simulink model "mech_transmission"  (Simulink 7.1)
settings: Solver=ode45  StartTime=0.0  StopTime=100  RelTol=1e-4  AbsTol=1e-4
PreLoadFcn:
  | load mech_transmission_data;
undefined symbols (not defined in the file or in its folder): converter_data, downtab, emap, Iei, Iint, mutable, Nf, r1, r2, radvec, thvec, uptab, vehicledata
libraries: mblibv1 x64
(part 1 of 2)
Description:
  | Automobile Transmission
  | 
  | Detailed model of an automotive gear box with Stateflow logic.
  | 
  | Stateflow is required only if you want to modify the existing logic charts.
settings Model: Creator=The MathWorks Inc.  ExtModeAutoUpdateStatusClock=off  BufferReuse=off
settings DataIOCC: SaveState=on  SignalLoggingName=sigsOut
settings OptimizationCC: BooleanDataType=off  InlineInvariantSignals=on  OptimizeBlockIOStorage=off  BufferReuse=off  ExpressionFolding=off  LocalBlockOutputs=off
settings DebuggingCC: AlgebraicLoopMsg=none  SaveWithParameterizedLinksMsg=none  CheckExecutionContextPreStartOutputMsg=on  CheckExecutionContextRuntimeOutputMsg=on  SignalResolutionControl=TryResolveAllWithWarning  SolverPrmCheckMsg=none  MultiTaskDSMMsg=warning  MultiTaskCondExecSysMsg=none  SigSpecEnsureSampleTimeMsg=none  StrictBusMsg=None
settings HardwareCC: TargetBitPerLong=64  TargetEndianess=LittleEndian  TargetWordSize=64  TargetHWDeviceType=MATLAB Host  ProdEqTarget=off
settings RTWCC: SystemTargetFile=rsim.tlc  TemplateMakefile=rsim_default_tmf  Description=Rapid Simulation Target  ProcessScript=rsim_make_rtw_hook  IncludeERTFirstTime=on
settings RSimTargetCC: TargetFcnLib=ansi_tfl_tmw.mat  TargetFunctionLibrary=ANSI_C  IsPILTarget=off  EnableShiftOperators=on  PortableWordSizes=off

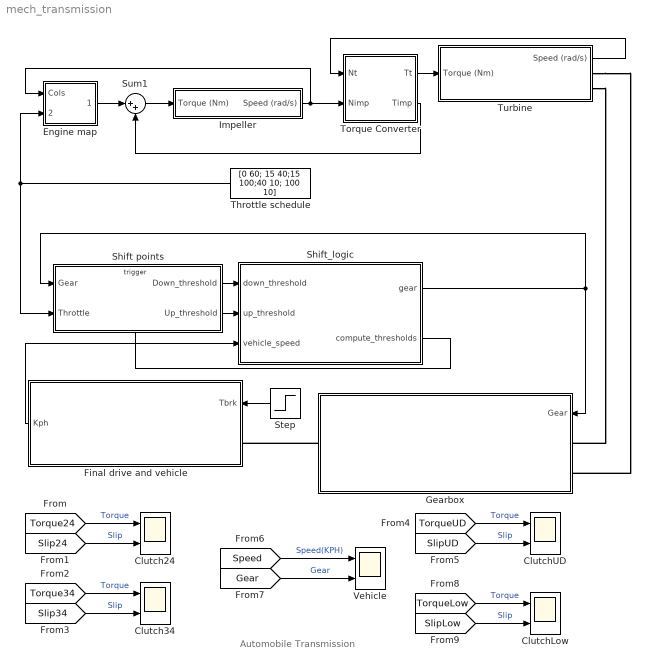
== system mech_transmission ==
  note: Automobile Transmission
  " Shift_logic" : Stateflow chart
  Clutch24 : Scope  NumInputPorts=2
      settings: TimeRange=100  YMin=-1000~-500  YMax=1000~500
  Clutch34 : Scope  NumInputPorts=2
      settings: TimeRange=100  YMin=-1000~-400  YMax=1000~200  SaveName=ScopeData2
  ClutchLow : Scope  NumInputPorts=2
      settings: TimeRange=100  YMin=-1000~0  YMax=500~600  SaveName=ScopeData4
  ClutchUD : Scope  NumInputPorts=2
      settings: TimeRange=100  YMin=-1000~-200  YMax=1000~400  SaveName=ScopeData3
  Engine map : Subsystem  AncestorBlock=|  mask(Lookup Table (2-D)){x=thvec, y=radvec, t=emap}
      | simulink3/Functions
      | & Tables/Look-Up
      | Table (2-D)
      mask prompts: x "Row:"; y "Column:"; t "Table:"
      mask help: Performs 2-D linear interpolation of input values using the specified input/output table. Extrapolation is performed outside the table boundaries. The first dimension corresponds to the top (or left) input port.
      mask init:
      | [r,c]=size(t);
      | xt=reshape(x,prod(size(x)),1);
      | xi=xt(:,ones(1,c));
      | minx=min(x); maxx=max(x);
      | mint=min(min(t)); maxt=max(max(t));
      mask Display: plot(double(xi),double(t),double([minx maxx]),double([mint mint]),double([minx minx]),double([mint maxt]))
  Final drive and vehicle : Subsystem  Orientation=left  mask(vehicle model){Rfd=vehicledata(1), rload0=vehicledata(2), rload2=vehicledata(3), Rw=vehicledata(4), inertiav=vehicledata(5), N20=vehicledata(6)/vehicledata(4)*vehicledata(1)}
      mask prompts: Rfd "Final drive ratio"; rload0 "Drag friction at wheels"; rload2 "Aerodynamic drag"; Rw "Wheel radius"; inertiav "Vehicle inertia"; N20 "Initial transmission output speed"
      mask help: vehicle dynamics: torque input from trans., outputs are input speed (transmission output) and vehicle speed
      mask Display: plot(-2,1,11,8,9-[cos(pi*[0:5:360]/180) + 6], [sin(pi*[0:5:360]/180) + 1.5],9-[cos(pi*[0:5:360]/180) + 1], [sin(pi*[0:5:360]/180) + 4],9- [10 7.5 6.75], [3.5 1 1.5], 9-[10 9.75 7.5 6.25 3 1.5 4 5 7.5], [3.5 4.75 5.5 7 8 7 6 4 5.5], 9-[6.5 4], [7 6],9- [5.25 2], [2 4],9- [7.5 1 0], [2.5 6 6.5],9- [7.5 7.25 9.75], [1 2.25 4.75],9- [2.75 2 0 0 0.25], [7.5 8 6.5 5.25 5],9- [1.5 0.5], [6.75 6.25])
  Gearbox : Subsystem  Orientation=left
      mask Display: plot(-5,-5,5,10,cos(0:.1:7),sin(0:.1:7),1.5*cos(0:.1:7),1.5*sin(0:.1:7)+3,[1.5 1],[3 0],[-1.5 -1],[3 0],0.5*cos(0:.1:7),0.5*sin(0:.1:7),cos(0:.1:7),sin(0:.1:7)+3)
  Impeller : Subsystem  mask{I=Iei, V=1.1}
      mask prompts: I "Impeller inertia (kg.m^2)"; V "Initial angular velocity (rad/s)"
  Shift points : Subsystem  TreatAsAtomicUnit=on
  Step : Step  Orientation=left  Time=60  After=380  SampleTime=0
  Sum1 : Sum  Inputs=|++  OutDataType=sfix(16)  OutScaling=2^0  SaturateOnIntegerOverflow=on
  Throttle schedule : FromWorkspace  Orientation=left  VariableName=[0 60; 15 40;15 100;40 10; 100 10]  SampleTime=0
  Torque Converter : Subsystem  mask(torque converter){speedratio=converter_data(:,1), Kfactor=converter_data(:,2), Torkratio=converter_data(:,3)}
      mask prompts: speedratio "speed ratio"; Kfactor "K factor"; Torkratio "torque ratio"
      mask help: torque converter
      mask Help: Torque converter input and output torques are computed as a function of the input and output speeds
      mask Display: plot([cos([90:10:450]*pi/180),.63*cos([90:10:450]*pi/180),.63*cos([90:10:240]*pi/180),cos([240:10:300]*pi/180),.63*cos([300]*pi/180)],[sin([90:10:450]*pi/180),.63*sin([90:10:450]*pi/180)+.1,.63*sin([90:10:240]*pi/180)+.1,sin([240:10:300]*pi/180),.63*sin([300]*pi/180)+.1])
  Turbine : Subsystem  mask{I=Iint, V=1}
      mask prompts: I "Turbine inertia (kg.m^2)"; V "Initial angular velocity (rad/s)"
  Vehicle : Scope  NumInputPorts=2
      settings: TimeRange=100  YMin=0~1  YMax=160~5
  wires:
  Sum1/1 -> Impeller/1(Torque (Nm))
  Impeller/1(Speed (rad/s)) -> Torque Converter/2(Nimp), Engine map/1(Cols)
  Torque Converter/1(Tt) -> Turbine/1(Torque (Nm))
  Engine map/1(Out1) -> Sum1/1
  Torque Converter/2(Timp) -> Sum1/2
  Turbine/1(Speed (rad/s)) -> Torque Converter/1(Nt)
  Shift points/2(Up_threshold) -> " Shift_logic"/2(up_threshold)
  Shift points/1(Down_threshold) -> " Shift_logic"/1(down_threshold)
  " Shift_logic"/2(compute_thresholds) -> Shift points/Trigger
  " Shift_logic"/1(gear) -> Shift points/1(Gear), Gearbox/1(Gear)
  Step/1 -> Final drive and vehicle/1(Tbrk)
  Final drive and vehicle/1(Kph) -> " Shift_logic"/3(vehicle_speed)
  [Torque24] -> Clutch24/1  "Torque"
  [Slip24] -> Clutch24/2  "Slip"
  [Torque34] -> Clutch34/1  "Torque"
  [Slip34] -> Clutch34/2  "Slip"
  [TorqueUD] -> ClutchUD/1  "Torque"
  [SlipUD] -> ClutchUD/2  "Slip"
  [Speed] -> Vehicle/1  "Speed(KPH)"
  [Gear] -> Vehicle/2  "Gear"
  [TorqueLow] -> ClutchLow/1  "Torque"
  [SlipLow] -> ClutchLow/2  "Slip"
  Throttle schedule/1 -> Engine map/2(Rows), Shift points/2(Throttle)
  connections:
  Turbine/RConn2 -- Gearbox/LConn1
  Turbine/RConn1 -- Gearbox/LConn2
  Gearbox/RConn1 -- Final drive and vehicle/LConn1

== system mech_transmission/Engine map ==
  Cols : Inport  OutDataType=sfix(16)  OutScaling=2^0
  Rows : Inport  Port=2  OutDataType=sfix(16)  OutScaling=2^0
  Look-Up Table (2-D) : Lookup2D  RowIndex=x  ColumnIndex=y  Table=t  OutDataType=sfix(16)  OutScaling=2^0  SaturateOnIntegerOverflow=on  InputSameDT=on
  Out1 : Outport  OutDataType=sfix(16)  OutScaling=2^0
  wires:
  Rows/1 -> Look-Up Table (2-D)/1
  Cols/1 -> Look-Up Table (2-D)/2
  Look-Up Table (2-D)/1 -> Out1/1

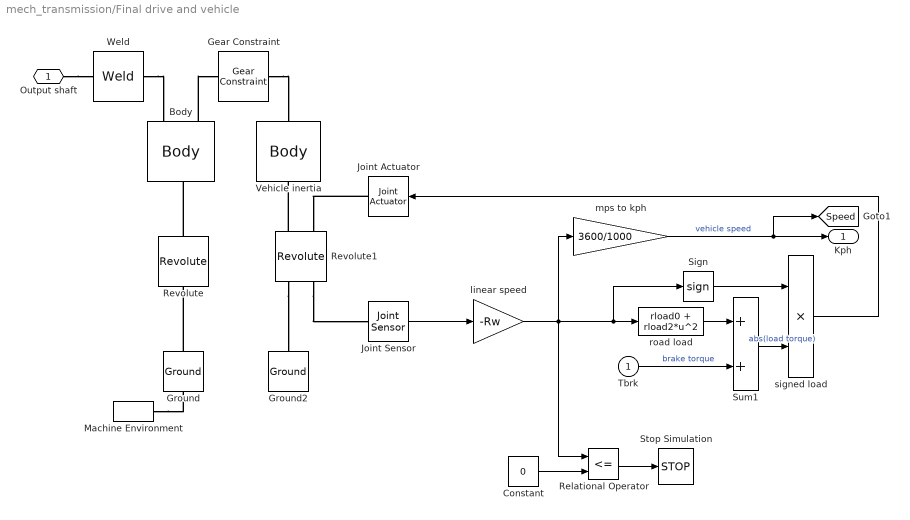
== system mech_transmission/Final drive and vehicle ==
  Tbrk : Inport  OutDataType=sfix(16)  OutScaling=2^0
  Body : mblibv1/Bodies/Body  Tag=Factory generic  Description=Mechanical Blockset  Orientation=down  DialogController=MECH.DynMechDlgSource  PhysicalDomain=mechanical  SubClassName=Unknown  LeftPortType=workingframe  RightPortType=workingframe  LConnTagsString=CS1|CS3  RConnTagsString=CS2  DialogClass=MechanicalBodyBlock  Mass=100  MassUnits=kg  InertiaUnits=kg*m^2  Inertia=diag([1e-4*0.5 1e-4*0.5 1e-4])  Shape=Cylinder  ShapeDims=[1 1]  ShapeUnits=m  ShapeUse=false  Density=1  DensityUnits=kg/m^3  DensityUse=false  GraphicsMode=1  BodyColor=[0.5 0.5 0.5]  GraphicsObj=[]  AttachedToCS=1  CG=Left$CG$[0 0 0]$WORLD$WORLD$m$[0 0 0]$Euler X-Y-Z$deg$WORLD$false  WorkingFrames=Left$CS1$[0 0 0]$CG$CG$m$[0 0 0]$Euler X-Y-Z$deg$WORLD$true#Left$CS3$[0 0 0]$CG$CG$m$[0 0 0]$Euler X-Y-Z$deg$WORLD$true#Right$CS2$[0 0 0]$CG$CG$m$[0 0 0]$Euler X-Y-Z$deg$WORLD$true  CGPos=[0 0 0]  CGRot=[0 0 0]  CS0Pos=[]  CS0Rot=[]  CS1Pos=[0 0 0]  CS1Rot=[0 0 0]  CS2Pos=[0 0 0]  CS2Rot=[0 0 0]  CS3Pos=[0 0 0]  CS3Rot=[0 0 0]  CS4Pos=[]  CS4Rot=[]  CS5Pos=[]  CS5Rot=[]  CS6Pos=[]  CS6Rot=[]  CS7Pos=[]  CS7Rot=[]  CS8Pos=[]  CS8Rot=[]  CS9Pos=[]  CS9Rot=[]  CS10Pos=[]  CS10Rot=[]  CS11Pos=[]  CS11Rot=[]  CS12Pos=[]  CS12Rot=[]  CS13Pos=[]  CS13Rot=[]  CS14Pos=[]  CS14Rot=[]  CS15Pos=[]  CS15Rot=[]  CS16Pos=[]  CS16Rot=[]  CS17Pos=[]  CS17Rot=[]  CS18Pos=[]  CS18Rot=[]  CS19Pos=[]  CS19Rot=[]  CS20Pos=[]  CS20Rot=[]
  Constant : Constant  Value=0  OutDataType=sfix(16)  OutScaling=2^0
  Gear Constraint : mblibv1/Constraints &  Drivers/Gear Constraint  Tag=Factory generic  Description=Mechanical Blockset  Orientation=left  DialogController=MECH.DynMechDlgSource  PhysicalDomain=mechanical  SubClassName=Unknown  LeftPortType=blob  RightPortType=blob  LConnTagsString=__newl0  RConnTagsString=__newr0  DialogClass=GearConstraint  NumSAPorts=0  BaseRadius=Rfd  BaseRadiusUnits=m  FollowerRadius=1  FollowerRadiusUnits=m
  Ground : mblibv1/Bodies/Ground  Orientation=up  DialogController=MECH.DynMechDlgSource  SystemSampleTime=-1  LeftPortType=env  RightPortType=workingframe  PhysicalDomain=Mechanical  DialogClass=GroundBlock  CoordPosition=[0 0 0]  CoordPositionUnits=m  StateVectorMgrId=-1  MachineId=[0 0]  ShowEnvPort=on
  Ground2 : mblibv1/Bodies/Ground  Orientation=up  DialogController=MECH.DynMechDlgSource  SystemSampleTime=-1  LeftPortType=env  RightPortType=workingframe  PhysicalDomain=Mechanical  DialogClass=GroundBlock  CoordPosition=[1+Rfd 0 0]  CoordPositionUnits=m  StateVectorMgrId=-1  MachineId=[0 0]  ShowEnvPort=off
  Joint Actuator : mblibv1/Sensors &  Actuators/Joint Actuator  Description=Mechanical Blockset  Orientation=left  DialogController=MECH.DynMechDlgSource  SystemSampleTime=-1  PhysicalDomain=Mechanical  PortType=blob  ActuationStyle=Force  AngleUnits=deg  ArcVelocityUnits=deg/s  ArcAccelerationUnits=deg/s^2  CoordPositionUnits=m  VelocityUnits=m/s  AccelerationUnits=m/s^2  ForceUnits=N  TorqueUnits=N-m  ActiveIO=on  Width=1  DialogClass=MechanicalActuatorBlock  Primitive=R1  ReferenceFrame=Absolute (INERTIAL)
  Joint Sensor : mblibv1/Sensors &  Actuators/Joint Sensor  Description=Mechanical Blockset  DialogController=MECH.DynMechDlgSource  SystemSampleTime=-1  PhysicalDomain=Mechanical  PortType=blob  Muxed=on  Pose=off  Angle=off  AngleUnits=deg  ArcVelocity=on  ArcVelocityUnits=rad/s  ArcAcceleration=off  ArcAccelerationUnits=deg/s^2  CoordPosition=on  CoordPositionUnits=m  Velocity=off  VelocityUnits=m/s  Acceleration=off  AccelerationUnits=m/s^2  Quaternion=on  QuaternionDT=off  QuaternionDDT=off  QuaternionUnits=off  OutputVector=[ 1 ]  ActiveIO=on  Width=1  DialogClass=MechanicalSensorBlock  Primitive=R1  Force=off  ForceUnits=N  Torque=off  TorqueUnits=N-m  ReferenceFrame=Absolute (INERTIAL)  ReactionSensedSide=Base  ReactionReferenceFrame=Absolute (World)  ReactionForce=off  ReactionForceUnits=N  ReactionMoment=off  ReactionMomentUnits=N-m
  Machine Environment : mblibv1/Bodies/Machine Environment  Tag=Factory ground  DialogController=MECH.DialogSource  SystemSampleTime=-1  PortType=env  PhysicalDomain=Mechanical  DialogTemplateClass=MECH.MachineEnvironment  SyncWhenCopied=off  Gravity=[0 -9.81 0]  GravityUnits=m/s^2  GravityAsSignal=off  Dimensionality=3D Only  AnalysisType=Forward dynamics  LinearAssemblyTolerance=1e-3  LinearAssemblyToleranceUnits=m  AngularAssemblyTolerance=1e-3  AngularAssemblyToleranceUnits=rad  ConstraintSolverType=Machine precision  ConstraintRelTolerance=1e-4  ConstraintAbsTolerance=1e-4  UseRobustSingularityHandling=off  RedundancyAnalysisToleranceType=Automatically select tolerance  RedundancyAnalysisTolerance=1e-14  StatePerturbationType=Fixed  PerturbationSize=1e-5  VisualizeMachine=on
  Relational Operator : RelationalOperator  Operator=<=
  Revolute : mblibv1/Joints/Revolute  Orientation=up  DialogController=MECH.DynMechDlgSource  PhysicalDomain=mechanical  SubClassName=Unknown  LeftPortType=blob  RightPortType=blob  LConnTagsString=__newl0  RConnTagsString=__newr0  NumSAPorts=0  CutJoint=off  MarkAsCut=off  Primitives=revolute  PrimitiveProps=R1$INERTIAL$[0 0 1]$revolute  DialogClass=JointBlock  R1Axis=[0 0 1]
  Revolute1 : mblibv1/Joints/Revolute  Orientation=up  DialogController=MECH.DynMechDlgSource  PhysicalDomain=mechanical  SubClassName=Unknown  LeftPortType=blob  RightPortType=blob  LConnTagsString=__newl0|SA1  RConnTagsString=__newr0|SA1  NumSAPorts=2  CutJoint=off  MarkAsCut=off  Primitives=revolute  PrimitiveProps=R1$WORLD$[0 0 1]$revolute  DialogClass=JointBlock  R1Axis=[0 0 1]
  Sign : Signum  ZeroCross=off
  Stop Simulation : Stop
  Sum1 : Sum  OutDataType=sfix(16)  OutScaling=2^0  SaturateOnIntegerOverflow=on  InputSameDT=on  OutDataTypeStr=Inherit: Same as first input
  Vehicle inertia : mblibv1/Bodies/Body  Tag=Factory generic  Description=Mechanical Blockset  Orientation=down  DialogController=MECH.DynMechDlgSource  PhysicalDomain=mechanical  SubClassName=Unknown  LeftPortType=workingframe  RightPortType=workingframe  LConnTagsString=CS1  RConnTagsString=CS2  DialogClass=MechanicalBodyBlock  Mass=200  MassUnits=kg  InertiaUnits=kg*m^2  Inertia=diag([inertiav*0.95 inertiav*0.1 inertiav])  Shape=Cylinder  ShapeDims=[1 1]  ShapeUnits=m  ShapeUse=false  Density=1  DensityUnits=kg/m^3  DensityUse=false  GraphicsMode=1  BodyColor=[0.5 0.5 0.5]  GraphicsObj=[]  AttachedToCS=1  CG=Left$CG$[1+Rfd 0 0]$WORLD$WORLD$m$[0 0 0]$Euler X-Y-Z$deg$WORLD$false  WorkingFrames=Left$CS1$[1+Rfd 0 0]$WORLD$WORLD$m$[0 0 0]$Euler X-Y-Z$deg$WORLD$true#Right$CS2$[1+Rfd 0 0]$WORLD$WORLD$m$[0 0 0]$Euler X-Y-Z$deg$WORLD$true  CGPos=[1+Rfd 0 0]  CGRot=[0 0 0]  CS0Pos=[]  CS0Rot=[]  CS1Pos=[1+Rfd 0 0]  CS1Rot=[0 0 0]  CS2Pos=[1+Rfd 0 0]  CS2Rot=[0 0 0]  CS3Pos=[]  CS3Rot=[]  CS4Pos=[]  CS4Rot=[]  CS5Pos=[]  CS5Rot=[]  CS6Pos=[]  CS6Rot=[]  CS7Pos=[]  CS7Rot=[]  CS8Pos=[]  CS8Rot=[]  CS9Pos=[]  CS9Rot=[]  CS10Pos=[]  CS10Rot=[]  CS11Pos=[]  CS11Rot=[]  CS12Pos=[]  CS12Rot=[]  CS13Pos=[]  CS13Rot=[]  CS14Pos=[]  CS14Rot=[]  CS15Pos=[]  CS15Rot=[]  CS16Pos=[]  CS16Rot=[]  CS17Pos=[]  CS17Rot=[]  CS18Pos=[]  CS18Rot=[]  CS19Pos=[]  CS19Rot=[]  CS20Pos=[]  CS20Rot=[]
  Weld : mblibv1/Joints/Weld  Orientation=left  DialogController=MECH.DynMechDlgSource  PhysicalDomain=mechanical  SubClassName=Unknown  LeftPortType=blob  RightPortType=blob  LConnTagsString=__newl0  RConnTagsString=__newr0  NumSAPorts=0  CutJoint=off  MarkAsCut=off  Primitives=weld  PrimitiveProps=W$INERTIAL$[0 0 0]$weld  DialogClass=JointBlock  WAxis=[0 0 0]
  linear speed : Gain  Gain=-Rw  ParameterDataType=sfix(16)  ParameterScaling=2^0  OutDataType=sfix(16)  OutScaling=2^0  SaturateOnIntegerOverflow=on  OutDataTypeStr=Inherit: Same as input  ParamDataTypeStr=Inherit: Same as input
  mps to kph : Gain  Gain=3600/1000  ParameterDataType=sfix(16)  ParameterScaling=2^0  OutDataType=sfix(16)  OutScaling=2^0  SaturateOnIntegerOverflow=on  OutDataTypeStr=Inherit: Same as input  ParamDataTypeStr=Inherit: Same as input
  road load : Fcn  Expr=rload0 + rload2*u^2
  signed load : Product  OutDataType=sfix(16)  OutScaling=2^0  SaturateOnIntegerOverflow=on  InputSameDT=on  OutDataTypeStr=Inherit: Same as first input
  Output shaft : PMIOPort  Port=1  Side=Left
  Kph : Outport  OutDataType=sfix(16)  OutScaling=2^0
  tag scope: Speed=global
  wires:
  mps to kph/1 -> Kph/1, [Speed]  "vehicle speed"
  Tbrk/1 -> Sum1/2  "brake torque"
  road load/1 -> Sum1/1
  Sign/1 -> signed load/1
  Sum1/1 -> signed load/2  "abs(load torque)"
  Joint Sensor/1 -> linear speed/1
  linear speed/1 -> mps to kph/1, Sign/1, road load/1, Relational Operator/1
  signed load/1 -> Joint Actuator/1
  Constant/1 -> Relational Operator/2
  Relational Operator/1 -> Stop Simulation/1
  connections:
  Ground/RConn1 -- Revolute/LConn1
  Revolute/RConn1 -- Body/RConn1
  Revolute1/LConn1 -- Ground2/RConn1
  Body/LConn2 -- Gear Constraint/RConn1
  Gear Constraint/LConn1 -- Vehicle inertia/LConn1
  Output shaft/RConn1 -- Weld/RConn1
  Weld/LConn1 -- Body/LConn1
  Revolute1/LConn2 -- Joint Sensor/LConn1
  Joint Actuator/RConn1 -- Revolute1/RConn2
  Revolute1/RConn1 -- Vehicle inertia/RConn1
  Machine Environment/RConn1 -- Ground/LConn1

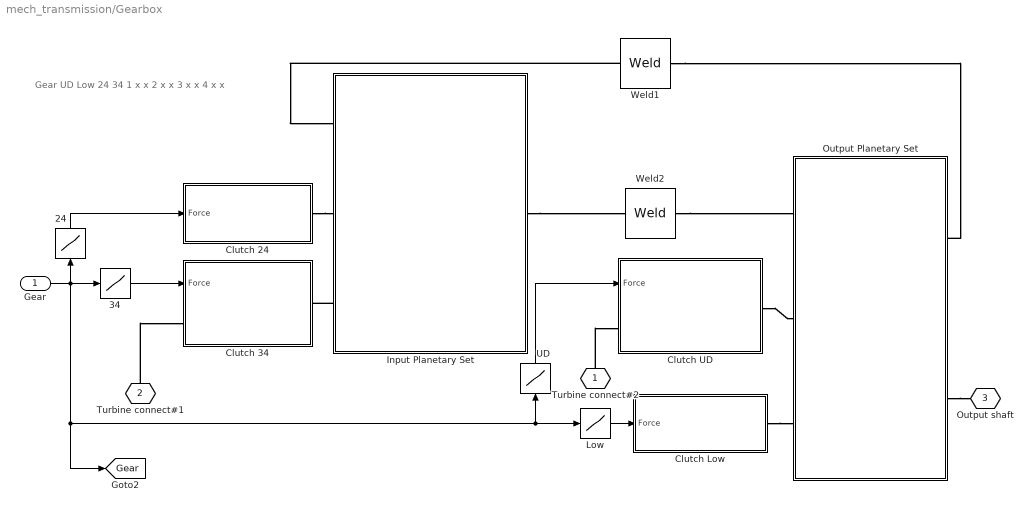
== system mech_transmission/Gearbox ==
  note: Gear   UD   Low   24   34
      | 1       x       x
      | 2       x               x
      |        3       x                        x
      |               4                        x       x
  Gear : Inport  OutDataType=sfix(16)  OutScaling=2^0
  24 : Lookup  Orientation=up  InputValues=[1 2 3 4]  Table=[0 1 0 1]*10e3  OutDataType=sfix(16)  OutScaling=2^0  SaturateOnIntegerOverflow=on
  34 : Lookup  InputValues=[1 2 3 4]  Table=[0 0 1 1]*10e3  OutDataType=sfix(16)  OutScaling=2^0  SaturateOnIntegerOverflow=on
  Clutch 24 : Subsystem  mask{rtq=2/3*(r2^3 - r1^3)/(r2^2 - r1^2), mutable=mutable, Nf=Nf}
      mask prompts: rtq "Effective torque radius"; mutable "Coefficient of friction table"; Nf "Number of friction surfaces"
      mask Display: plot(-1,-2,6,8,[0 3],[3 3],[3 1 1 3], [1 1 5 5],[2 4 4 2],[4 4 2 2],[4 5],[3 3])
  Clutch 34 : Subsystem  mask{rtq=2/3*(r2^3 - r1^3)/(r2^2 - r1^2), mutable=mutable, Nf=Nf}
      mask prompts: rtq "Effective torque radius"; mutable "Coefficient of friction table"; Nf "Number of friction surfaces"
      mask Display: plot(-1,-2,6,8,[0 3],[3 3],[3 1 1 3], [1 1 5 5],[2 4 4 2],[4 4 2 2],[4 5],[3 3])
  Clutch Low : Subsystem  mask{rtq=2/3*(r2^3 - r1^3)/(r2^2 - r1^2), mutable=mutable, Nf=Nf}
      mask prompts: rtq "Effective torque radius"; mutable "Coefficient of friction table"; Nf "Number of friction surfaces"
      mask Display: plot(-1,-2,6,8,[0 3],[3 3],[3 1 1 3], [1 1 5 5],[2 4 4 2],[4 4 2 2],[4 5],[3 3])
  Clutch UD : Subsystem  mask{rtq=2/3*(r2^3 - r1^3)/(r2^2 - r1^2), mutable=mutable, Nf=Nf}
      mask prompts: rtq "Effective torque radius"; mutable "Coefficient of friction table"; Nf "Number of friction surfaces"
      mask Display: plot(-1,-2,6,8,[0 3],[3 3],[3 1 1 3], [1 1 5 5],[2 4 4 2],[4 4 2 2],[4 5],[3 3])
  Input Planetary Set : Subsystem  Orientation=left  mask{R=2.0960, Is=1e-4, Ir=1e-4, Ic=1e-4, Ip=1e-6}
      mask prompts: R "Ring/Sun tooth ratio"; Is "Sun inertia (kg*m^2)"; Ir "Ring inertia (kg*m^2)"; Ic "Carrier inertia (kg*m^2)"; Ip "Total planet inertia (kg*m^2)"
      mask Display: plot(-2,-4,2,6,cos(0:.1:2*pi),sin(0:.1:2*pi),1.6*cos(0:.1:2*pi),1.6*sin(0:.1:2*pi),.3*cos(0:.1:2*pi)-1.3,.3*sin(0:.1:2*pi),.3*cos(0:.1:2*pi)+1.3,.3*sin(0:.1:2*pi),.3*cos(0:.1:2*pi),.3*sin(0:.1:2*pi)+1.3,.3*cos(0:.1:2*pi),.3*sin(0:.1:2*pi)-1.3)
  Low : Lookup  InputValues=[1 2 3 4]  Table=[1 0 0 0]*10e3  OutDataType=sfix(16)  OutScaling=2^0  SaturateOnIntegerOverflow=on
  Output Planetary Set : Subsystem  Orientation=left  mask{R=1.3930, Is=1e-4, Ir=1e-4, Ic=1e-4, Ip=1e-6}
      mask prompts: R "Ring/Sun tooth ratio"; Is "Sun inertia (kg*m^2)"; Ir "Ring inertia (kg*m^2)"; Ic "Carrier inertia (kg*m^2)"; Ip "Total planet inertia (kg*m^2)"
      mask Display: plot(-2,-4,2,6,cos(0:.1:2*pi),sin(0:.1:2*pi),1.6*cos(0:.1:2*pi),1.6*sin(0:.1:2*pi),.3*cos(0:.1:2*pi)-1.3,.3*sin(0:.1:2*pi),.3*cos(0:.1:2*pi)+1.3,.3*sin(0:.1:2*pi),.3*cos(0:.1:2*pi),.3*sin(0:.1:2*pi)+1.3,.3*cos(0:.1:2*pi),.3*sin(0:.1:2*pi)-1.3)
  UD : Lookup  Orientation=up  InputValues=[1 2 3 4]  Table=[1 1 1 0]*10e3  OutDataType=sfix(16)  OutScaling=2^0  SaturateOnIntegerOverflow=on
  Weld1 : mblibv1/Joints/Weld  Tag=Factory generic  Description=Mechanical Blockset  DialogController=MECH.DynMechDlgSource  PhysicalDomain=mechanical  SubClassName=Unknown  LeftPortType=blob  RightPortType=blob  LConnTagsString=__newl0  RConnTagsString=__newr0  NumSAPorts=0  CutJoint=on  MarkAsCut=off  Primitives=weld  PrimitiveProps=W$WORLD$[0 0 0]$weld  DialogClass=JointBlock  WAxis=[0 0 0]
  Weld2 : mblibv1/Joints/Weld  Tag=Factory generic  Description=Mechanical Blockset  DialogController=MECH.DynMechDlgSource  PhysicalDomain=mechanical  SubClassName=Unknown  LeftPortType=blob  RightPortType=blob  LConnTagsString=__newl0  RConnTagsString=__newr0  NumSAPorts=0  CutJoint=on  MarkAsCut=off  Primitives=weld  PrimitiveProps=W$WORLD$[0 0 0]$weld  DialogClass=JointBlock  WAxis=[0 0 0]
  Turbine connect#2 : PMIOPort  Tag=PMCPort  Orientation=up  Port=1  Side=Left
  Turbine connect#1 : PMIOPort  Tag=PMCPort  Orientation=up  Port=2  Side=Left
  Output shaft : PMIOPort  Tag=PMCPort  Orientation=left  Port=3  Side=Right
  tag scope: Gear=global
  wires:
  UD/1 -> Clutch UD/1(Force)
  Low/1 -> Clutch Low/1(Force)
  24/1 -> Clutch 24/1(Force)
  34/1 -> Clutch 34/1(Force)
  Gear/1 -> 34/1, 24/1, Low/1, UD/1, [Gear]
  connections:
  Clutch UD/RConn1 -- Output Planetary Set/RConn2
  Clutch 24/RConn1 -- Input Planetary Set/RConn2
  Input Planetary Set/RConn3 -- Clutch 34/RConn1
  Weld2/RConn1 -- Output Planetary Set/RConn1
  Weld1/RConn1 -- Output Planetary Set/LConn1
  Clutch Low/RConn1 -- Output Planetary Set/RConn3
  Output Planetary Set/LConn2 -- Output shaft/RConn1
  Weld1/LConn1 -- Input Planetary Set/RConn1
  Input Planetary Set/LConn1 -- Weld2/LConn1
  Turbine connect#1/RConn1 -- Clutch 34/LConn1
  Turbine connect#2/RConn1 -- Clutch UD/LConn1

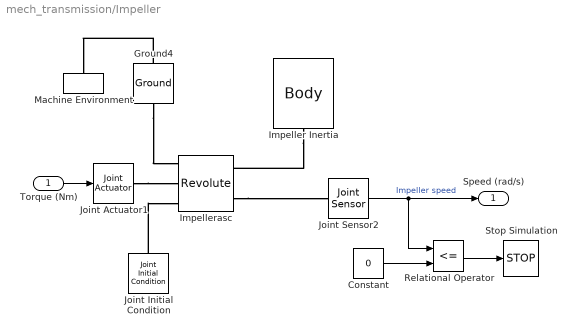
== system mech_transmission/Impeller ==
  Torque (Nm) : Inport  OutDataType=sfix(16)  OutScaling=2^0
  Constant : Constant  Value=0  OutDataType=sfix(16)  OutScaling=2^0
  Ground4 : mblibv1/Bodies/Ground  Orientation=down  DialogController=MECH.DynMechDlgSource  SystemSampleTime=-1  LeftPortType=env  RightPortType=workingframe  PhysicalDomain=Mechanical  DialogClass=GroundBlock  CoordPosition=[0 0 0]  CoordPositionUnits=m  StateVectorMgrId=-1  MachineId=[0 0]  ShowEnvPort=on
  Impeller Inertia : mblibv1/Bodies/Body  Tag=Factory generic  Description=Mechanical Blockset  Orientation=up  DialogController=MECH.DynMechDlgSource  PhysicalDomain=mechanical  SubClassName=Unknown  LeftPortType=workingframe  RightPortType=workingframe  LConnTagsString=CS1  DialogClass=MechanicalBodyBlock  Mass=0.1  MassUnits=kg  InertiaUnits=kg*m^2  Inertia=diag([I*0.501 I*0.501 I])  Shape=Cylinder  ShapeDims=[1 1]  ShapeUnits=m  ShapeUse=false  Density=1  DensityUnits=kg/m^3  DensityUse=false  GraphicsMode=1  BodyColor=[0.5 0.5 0.5]  GraphicsObj=[]  AttachedToCS=1  CG=Left$CG$[0 0 -1]$WORLD$WORLD$m$[0 0 0]$Euler X-Y-Z$deg$WORLD$false  WorkingFrames=Left$CS1$[0 0 0]$WORLD$WORLD$m$[0 0 0]$Euler X-Y-Z$deg$WORLD$true  CGPos=[0 0 -1]  CGRot=[0 0 0]  CS0Pos=[]  CS0Rot=[]  CS1Pos=[0 0 0]  CS1Rot=[0 0 0]  CS2Pos=[]  CS2Rot=[]  CS3Pos=[]  CS3Rot=[]  CS4Pos=[]  CS4Rot=[]  CS5Pos=[]  CS5Rot=[]  CS6Pos=[]  CS6Rot=[]  CS7Pos=[]  CS7Rot=[]  CS8Pos=[]  CS8Rot=[]  CS9Pos=[]  CS9Rot=[]  CS10Pos=[]  CS10Rot=[]  CS11Pos=[]  CS11Rot=[]  CS12Pos=[]  CS12Rot=[]  CS13Pos=[]  CS13Rot=[]  CS14Pos=[]  CS14Rot=[]  CS15Pos=[]  CS15Rot=[]  CS16Pos=[]  CS16Rot=[]  CS17Pos=[]  CS17Rot=[]  CS18Pos=[]  CS18Rot=[]  CS19Pos=[]  CS19Rot=[]  CS20Pos=[]  CS20Rot=[]
  Impellerasc : mblibv1/Joints/Revolute  Tag=Factory generic  Description=Mechanical Blockset  DialogController=MECH.DynMechDlgSource  PhysicalDomain=mechanical  SubClassName=Unknown  LeftPortType=blob  RightPortType=blob  LConnTagsString=__newl0|SA1|SA2  RConnTagsString=__newr0|SA1  NumSAPorts=3  CutJoint=off  MarkAsCut=off  Primitives=revolute  PrimitiveProps=R1$WORLD$[0 0 1]$revolute  DialogClass=JointBlock  R1Axis=[0 0 1]
  Joint Actuator1 : mblibv1/Sensors &  Actuators/Joint Actuator  Description=Mechanical Blockset  DialogController=MECH.DynMechDlgSource  SystemSampleTime=-1  PhysicalDomain=Mechanical  PortType=blob  ActuationStyle=Force  AngleUnits=rad  ArcVelocityUnits=rad/s  ArcAccelerationUnits=rad/s^2  CoordPositionUnits=m  VelocityUnits=m/s  AccelerationUnits=m/s^2  ForceUnits=N  TorqueUnits=N-m  ActiveIO=on  Width=1  DialogClass=MechanicalActuatorBlock  Primitive=R1  ReferenceFrame=Absolute (INERTIAL)
  Joint Initial Condition : mblibv1/Sensors &  Actuators/Joint Initial Condition  Description=Mechanical Blockset  Orientation=up  DialogController=MECH.DynMechDlgSource  SystemSampleTime=-1  PhysicalDomain=Mechanical  DialogClass=InitialConditionBlock  Primitive=R1  CoordPosition=0.0  Velocity=V  AngleUnits=rad  ArcVelocityUnits=rad/s  CoordPositionUnits=m  VelocityUnits=m/s  InitialConditions=P1$false$0$m$rad$0$m/s$rad/s#P2$false$0$m$rad$0$m/s$rad/s#P3$false$0$m$rad$0$m/s$rad/s#R1$true$0.0$m$rad$V$m/s$rad/s#R2$false$0$m$rad$0$m/s$rad/s#R3$false$0$m$rad$0$m/s$rad/s#S$false$0$m$rad$0$m/s$rad/s  P1PIC=0  P1VIC=0  P2PIC=0  P2VIC=0  P3PIC=0  P3VIC=0  R1PIC=0.0  R1VIC=V  R2PIC=0  R2VIC=0  R3PIC=0  R3VIC=0  SPIC=0  SVIC=0
  Joint Sensor2 : mblibv1/Sensors &  Actuators/Joint Sensor  Description=Mechanical Blockset  DialogController=MECH.DynMechDlgSource  SystemSampleTime=-1  PhysicalDomain=Mechanical  PortType=blob  Muxed=off  Pose=off  Angle=off  AngleUnits=deg  ArcVelocity=on  ArcVelocityUnits=rad/s  ArcAcceleration=off  ArcAccelerationUnits=deg/s^2  CoordPosition=on  CoordPositionUnits=m  Velocity=off  VelocityUnits=m/s  Acceleration=off  AccelerationUnits=m/s^2  Quaternion=on  QuaternionDT=off  QuaternionDDT=off  QuaternionUnits=off  OutputVector=[ 1 ]  ActiveIO=on  Width=1  DialogClass=MechanicalSensorBlock  Primitive=R1  Force=off  ForceUnits=N  Torque=off  TorqueUnits=N-m  ReferenceFrame=Absolute (INERTIAL)  ReactionSensedSide=Base  ReactionReferenceFrame=Absolute (World)  ReactionForce=off  ReactionForceUnits=N  ReactionMoment=off  ReactionMomentUnits=N-m
  Machine Environment : mblibv1/Bodies/Machine Environment  Tag=Factory ground  Orientation=up  DialogController=MECH.DialogSource  SystemSampleTime=-1  PortType=env  PhysicalDomain=Mechanical  DialogTemplateClass=MECH.MachineEnvironment  SyncWhenCopied=off  Gravity=[0 -9.81 0]  GravityUnits=m/s^2  GravityAsSignal=off  Dimensionality=3D Only  AnalysisType=Forward dynamics  LinearAssemblyTolerance=1e-3  LinearAssemblyToleranceUnits=m  AngularAssemblyTolerance=1e-3  AngularAssemblyToleranceUnits=rad  ConstraintSolverType=Machine precision  ConstraintRelTolerance=1e-4  ConstraintAbsTolerance=1e-4  UseRobustSingularityHandling=off  RedundancyAnalysisToleranceType=Automatically select tolerance  RedundancyAnalysisTolerance=1e-14  StatePerturbationType=Fixed  PerturbationSize=1e-5  VisualizeMachine=on
  Relational Operator : RelationalOperator  Operator=<=
  Stop Simulation : Stop
  Speed (rad/s) : Outport  OutDataType=sfix(16)  OutScaling=2^0
  wires:
  Torque (Nm)/1 -> Joint Actuator1/1
  Joint Sensor2/1 -> Speed (rad/s)/1, Relational Operator/1  "Impeller speed"
  Constant/1 -> Relational Operator/2
  Relational Operator/1 -> Stop Simulation/1
  connections:
  Ground4/RConn1 -- Impellerasc/LConn1
  Impeller Inertia/LConn1 -- Impellerasc/RConn1
  Joint Actuator1/RConn1 -- Impellerasc/LConn2
  Joint Initial Condition/RConn1 -- Impellerasc/LConn3
  Impellerasc/RConn2 -- Joint Sensor2/LConn1
  Ground4/LConn1 -- Machine Environment/RConn1

== system mech_transmission/Shift points ==
  Gear : Inport  OutDataType=sfix(16)  OutScaling=2^0
  Throttle : Inport  Port=2  OutDataType=sfix(16)  OutScaling=2^0
  ev : TriggerPort  TriggerType=function-call  ZeroCross=off
  downshifts : Lookup2D  RowIndex=downth  ColumnIndex=[1 2 3 4]  Table=downtab  OutDataType=sfix(16)  OutScaling=2^0  SaturateOnIntegerOverflow=on  InputSameDT=on
  upshifts : Lookup2D  RowIndex=upth  ColumnIndex=[1 2 3 4]  Table=uptab  OutDataType=sfix(16)  OutScaling=2^0  SaturateOnIntegerOverflow=on  InputSameDT=on
  Down_threshold : Outport  OutDataType=sfix(16)  OutScaling=2^0  InitialOutput=0
  Up_threshold : Outport  Port=2  OutDataType=sfix(16)  OutScaling=2^0  InitialOutput=0
  wires:
  Gear/1 -> upshifts/2, downshifts/2
  Throttle/1 -> upshifts/1, downshifts/1
  upshifts/1 -> Up_threshold/1
  downshifts/1 -> Down_threshold/1

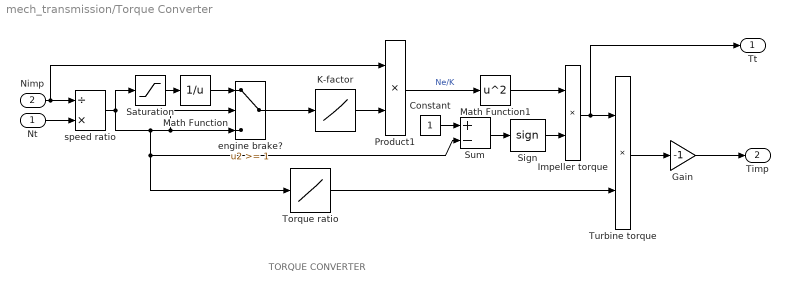
== system mech_transmission/Torque Converter ==
  note: TORQUE CONVERTER
  Nt : Inport  OutDataType=sfix(16)  OutScaling=2^0
  Nimp : Inport  Port=2  OutDataType=sfix(16)  OutScaling=2^0
  Constant : Constant  OutDataType=sfix(16)  OutScaling=2^0
  Gain : Gain  Gain=-1  ParameterDataType=sfix(16)  ParameterScaling=2^0  OutDataType=sfix(16)  OutScaling=2^0  SaturateOnIntegerOverflow=on  OutDataTypeStr=Inherit: Same as input  ParamDataTypeStr=Inherit: Same as input
  Impeller torque : Product  OutDataType=sfix(16)  OutScaling=2^0  SaturateOnIntegerOverflow=on  InputSameDT=on  OutDataTypeStr=Inherit: Same as first input
  K-factor : Lookup  InputValues=speedratio  Table=Kfactor  OutDataType=sfix(16)  OutScaling=2^0  SaturateOnIntegerOverflow=on
  Math Function : Math  Operator=reciprocal  OutDataType=sfix(16)  OutScaling=2^0  SaturateOnIntegerOverflow=on
  Math Function1 : Math  Operator=square  OutDataType=sfix(16)  OutScaling=2^0  SaturateOnIntegerOverflow=on
  Product1 : Product  Inputs=**  OutDataType=sfix(16)  OutScaling=2^0  SaturateOnIntegerOverflow=on  InputSameDT=on  OutDataTypeStr=Inherit: Same as first input
  Saturation : Saturate  UpperLimit=Inf  LowerLimit=1  ZeroCross=off
  Sign : Signum  ZeroCross=off
  Sum : Sum  Inputs=+-  OutDataType=sfix(16)  OutScaling=2^0  SaturateOnIntegerOverflow=on  InputSameDT=on  OutDataTypeStr=Inherit: Same as first input
  Torque ratio : Lookup  InputValues=speedratio  Table=Torkratio  OutDataType=sfix(16)  OutScaling=2^0  SaturateOnIntegerOverflow=on
  Turbine torque : Product  OutDataType=sfix(16)  OutScaling=2^0  SaturateOnIntegerOverflow=on  InputSameDT=on  OutDataTypeStr=Inherit: Same as first input
  engine brake? : Switch  Threshold=1  ZeroCross=off  InputSameDT=on
  speed ratio : Product  Inputs=/*  OutDataType=sfix(16)  OutScaling=2^0  SaturateOnIntegerOverflow=on  InputSameDT=on  OutDataTypeStr=Inherit: Same as first input
  Tt : Outport  OutDataType=sfix(16)  OutScaling=2^0  InitialOutput=0
  Timp : Outport  Port=2  OutDataType=sfix(16)  OutScaling=2^0  InitialOutput=0
  wires:
  Saturation/1 -> Math Function/1
  Math Function/1 -> engine brake?/1
  engine brake?/1 -> K-factor/1
  speed ratio/1 -> Saturation/1, engine brake?/2, engine brake?/3, Sum/2, Torque ratio/1
  Constant/1 -> Sum/1
  Sum/1 -> Sign/1
  Impeller torque/1 -> Turbine torque/1, Tt/1
  Math Function1/1 -> Impeller torque/1
  Sign/1 -> Impeller torque/2
  Product1/1 -> Math Function1/1  "Ne/K"
  Torque ratio/1 -> Turbine torque/2
  K-factor/1 -> Product1/2
  Turbine torque/1 -> Gain/1
  Nimp/1 -> speed ratio/1, Product1/1
  Nt/1 -> speed ratio/2
  Gain/1 -> Timp/1

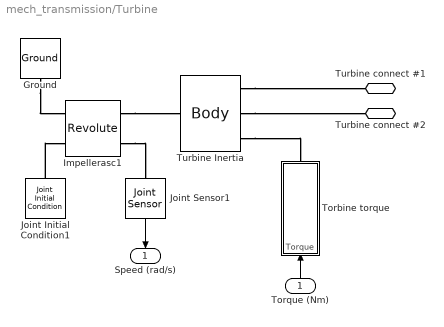
== system mech_transmission/Turbine ==
  Torque (Nm) : Inport  Orientation=up  OutDataType=sfix(16)  OutScaling=2^0
  Ground : mblibv1/Bodies/Ground  Orientation=down  DialogController=MECH.DynMechDlgSource  SystemSampleTime=-1  LeftPortType=env  RightPortType=workingframe  PhysicalDomain=Mechanical  DialogClass=GroundBlock  CoordPosition=[0 0 0]  CoordPositionUnits=m  StateVectorMgrId=-1  MachineId=[0 0]  ShowEnvPort=off
  Impellerasc1 : mblibv1/Joints/Revolute  Tag=Factory generic  Description=Mechanical Blockset  DialogController=MECH.DynMechDlgSource  PhysicalDomain=mechanical  SubClassName=Unknown  LeftPortType=blob  RightPortType=blob  LConnTagsString=__newl0|SA1  RConnTagsString=__newr0|SA1  NumSAPorts=2  CutJoint=off  MarkAsCut=off  Primitives=revolute  PrimitiveProps=R1$WORLD$[0 0 1]$revolute  DialogClass=JointBlock  R1Axis=[0 0 1]
  Joint Initial Condition1 : mblibv1/Sensors &  Actuators/Joint Initial Condition  Description=Mechanical Blockset  Orientation=up  DialogController=MECH.DynMechDlgSource  SystemSampleTime=-1  PhysicalDomain=Mechanical  DialogClass=InitialConditionBlock  Primitive=R1  CoordPosition=0.0  Velocity=V  AngleUnits=rad  ArcVelocityUnits=rad/s  CoordPositionUnits=m  VelocityUnits=m/s  InitialConditions=P1$false$0$m$rad$0$m/s$rad/s#P2$false$0$m$rad$0$m/s$rad/s#P3$false$0$m$rad$0$m/s$rad/s#R1$true$0.0$m$rad$V$m/s$rad/s#R2$false$0$m$rad$0$m/s$rad/s#R3$false$0$m$rad$0$m/s$rad/s#S$false$0$m$rad$0$m/s$rad/s  P1PIC=0  P1VIC=0  P2PIC=0  P2VIC=0  P3PIC=0  P3VIC=0  R1PIC=0.0  R1VIC=V  R2PIC=0  R2VIC=0  R3PIC=0  R3VIC=0  SPIC=0  SVIC=0
  Joint Sensor1 : mblibv1/Sensors &  Actuators/Joint Sensor  Description=Mechanical Blockset  Orientation=down  DialogController=MECH.DynMechDlgSource  SystemSampleTime=-1  PhysicalDomain=Mechanical  PortType=blob  Muxed=off  Pose=off  Angle=off  AngleUnits=deg  ArcVelocity=on  ArcVelocityUnits=rad/s  ArcAcceleration=off  ArcAccelerationUnits=deg/s^2  CoordPosition=on  CoordPositionUnits=m  Velocity=off  VelocityUnits=m/s  Acceleration=off  AccelerationUnits=m/s^2  Quaternion=on  QuaternionDT=off  QuaternionDDT=off  QuaternionUnits=off  OutputVector=[ 1 ]  ActiveIO=on  Width=1  DialogClass=MechanicalSensorBlock  Primitive=R1  Force=off  ForceUnits=N  Torque=off  TorqueUnits=N-m  ReferenceFrame=Absolute (INERTIAL)  ReactionSensedSide=Base  ReactionReferenceFrame=Absolute (World)  ReactionForce=off  ReactionForceUnits=N  ReactionMoment=off  ReactionMomentUnits=N-m
  Torbine torque : Subsystem  Orientation=up
  Turbine Inertia : mblibv1/Bodies/Body  Tag=Factory generic  Description=Mechanical Blockset  DialogController=MECH.DynMechDlgSource  PhysicalDomain=mechanical  SubClassName=Unknown  LeftPortType=workingframe  RightPortType=workingframe  LConnTagsString=CS1  RConnTagsString=CS2|CS4|CS3  DialogClass=MechanicalBodyBlock  Mass=5  MassUnits=g  InertiaUnits=kg*m^2  Inertia=diag([I*0.501 I*0.501 I])  Shape=Cylinder  ShapeDims=[1 1]  ShapeUnits=m  ShapeUse=false  Density=1  DensityUnits=kg/m^3  DensityUse=false  GraphicsMode=1  BodyColor=[0.5 0.5 0.5]  GraphicsObj=[]  AttachedToCS=1  CG=Left$CG$[0 0 -1.5]$WORLD$WORLD$m$[0 0 0]$Euler X-Y-Z$deg$WORLD$false  WorkingFrames=Left$CS1$[0 0 0]$WORLD$WORLD$m$[0 0 0]$Euler X-Y-Z$deg$WORLD$true#Right$CS2$[0 0 0]$CS1$CS1$m$[0 0 0]$Euler X-Y-Z$deg$WORLD$true#Right$CS4$[0 0 0]$CS1$CS1$m$[0 0 0]$Euler X-Y-Z$deg$WORLD$true#Right$CS3$[0 0 0]$CS1$CS1$m$[0 0 0]$Euler X-Y-Z$deg$WORLD$true  CGPos=[0 0 -1.5]  CGRot=[0 0 0]  CS0Pos=[]  CS0Rot=[]  CS1Pos=[0 0 0]  CS1Rot=[0 0 0]  CS2Pos=[0 0 0]  CS2Rot=[0 0 0]  CS3Pos=[0 0 0]  CS3Rot=[0 0 0]  CS4Pos=[0 0 0]  CS4Rot=[0 0 0]  CS5Pos=[]  CS5Rot=[]  CS6Pos=[]  CS6Rot=[]  CS7Pos=[]  CS7Rot=[]  CS8Pos=[]  CS8Rot=[]  CS9Pos=[]  CS9Rot=[]  CS10Pos=[]  CS10Rot=[]  CS11Pos=[]  CS11Rot=[]  CS12Pos=[]  CS12Rot=[]  CS13Pos=[]  CS13Rot=[]  CS14Pos=[]  CS14Rot=[]  CS15Pos=[]  CS15Rot=[]  CS16Pos=[]  CS16Rot=[]  CS17Pos=[]  CS17Rot=[]  CS18Pos=[]  CS18Rot=[]  CS19Pos=[]  CS19Rot=[]  CS20Pos=[]  CS20Rot=[]
  Turbine connect #1 : PMIOPort  Tag=PMCPort  Orientation=left  Port=1  Side=Right
  Turbine connect #2 : PMIOPort  Tag=PMCPort  Orientation=left  Port=2  Side=Right
  Speed (rad/s) : Outport  Orientation=down  OutDataType=sfix(16)  OutScaling=2^0
  wires:
  Joint Sensor1/1 -> Speed (rad/s)/1
  Torque (Nm)/1 -> Torbine torque/1(Torque)
  connections:
  Impellerasc1/RConn1 -- Turbine Inertia/LConn1
  Turbine Inertia/RConn3 -- Torbine torque/RConn1
  Turbine Inertia/RConn1 -- Turbine connect #1/RConn1
  Turbine Inertia/RConn2 -- Turbine connect #2/RConn1
  Ground/RConn1 -- Impellerasc1/LConn1
  Joint Initial Condition1/RConn1 -- Impellerasc1/LConn2
  Impellerasc1/RConn2 -- Joint Sensor1/LConn1

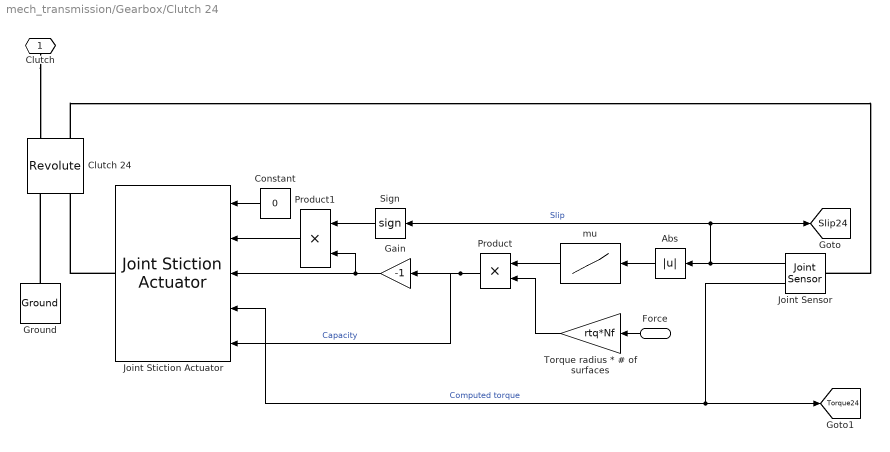
== system mech_transmission/Gearbox/Clutch 24 ==
  Force : Inport  Orientation=left  OutDataType=sfix(16)  OutScaling=2^0
  Abs : Abs  Orientation=left  ZeroCross=off  SaturateOnIntegerOverflow=on
  Clutch 24 : mblibv1/Joints/Revolute  Tag=Factory generic  Description=Mechanical Blockset  Orientation=up  DialogController=MECH.DynMechDlgSource  PhysicalDomain=mechanical  SubClassName=Unknown  LeftPortType=blob  RightPortType=blob  LConnTagsString=__newl0|SA1  RConnTagsString=__newr0|SA1  NumSAPorts=2  CutJoint=on  MarkAsCut=off  Primitives=revolute  PrimitiveProps=R1$WORLD$[0 0 1]$revolute  DialogClass=JointBlock  R1Axis=[0 0 1]
  Constant : Constant  Orientation=left  Value=0  OutDataType=sfix(16)  OutScaling=2^0
  Gain : Gain  Orientation=left  Gain=-1  ParameterDataType=sfix(16)  ParameterScaling=2^0  OutDataType=sfix(16)  OutScaling=2^0  SaturateOnIntegerOverflow=on  OutDataTypeStr=Inherit: Same as input  ParamDataTypeStr=Inherit: Same as input
  Ground : mblibv1/Bodies/Ground  Orientation=up  DialogController=MECH.DynMechDlgSource  SystemSampleTime=-1  LeftPortType=env  RightPortType=workingframe  PhysicalDomain=Mechanical  DialogClass=GroundBlock  CoordPosition=[0 0 0]  CoordPositionUnits=m  StateVectorMgrId=-1  MachineId=[0 0]  ShowEnvPort=off
  Joint Sensor : mblibv1/Sensors &  Actuators/Joint Sensor  Description=Mechanical Blockset  Orientation=left  DialogController=MECH.DynMechDlgSource  SystemSampleTime=-1  PhysicalDomain=Mechanical  PortType=blob  Muxed=off  Pose=off  Angle=off  AngleUnits=deg  ArcVelocity=on  ArcVelocityUnits=rad/s  ArcAcceleration=off  ArcAccelerationUnits=deg/s^2  CoordPosition=on  CoordPositionUnits=m  Velocity=off  VelocityUnits=m/s  Acceleration=off  AccelerationUnits=m/s^2  Quaternion=on  QuaternionDT=off  QuaternionDDT=off  QuaternionUnits=off  OutputVector=[ 1 1 ]  ActiveIO=on  Width=2  DialogClass=MechanicalSensorBlock  Primitive=R1  Force=off  ForceUnits=N  Torque=on  TorqueUnits=N-m  ReferenceFrame=Absolute (INERTIAL)  ReactionSensedSide=Base  ReactionReferenceFrame=Absolute (World)  ReactionForce=off  ReactionForceUnits=N  ReactionMoment=off  ReactionMomentUnits=N-m
  Joint Stiction Actuator : mblibv1/Sensors &  Actuators/Joint Stiction Actuator  Description=Mechanical Blockset  Orientation=left  DialogController=MECH.DynMechDlgSource  SystemSampleTime=-1  PhysicalDomain=Mechanical  PortType=blob  ActuationStyle=Force  AngleUnits=deg  ArcVelocityUnits=deg/s  ArcAccelerationUnits=deg/s^2  CoordPositionUnits=m  VelocityUnits=m/s  AccelerationUnits=m/s^2  ForceUnits=N  TorqueUnits=N-m  ActiveIO=on  Width=5  DialogClass=EventActuatorBlock  Primitive=R1  FrictionalForceUnits=N-m  ExternalForceUnits=N-m  FrictionalTorqueUnits=N-m  ExternalTorqueUnits=N-m  LockingTolerance=1e-3
  Product : Product  Orientation=left  OutDataType=sfix(16)  OutScaling=2^0  SaturateOnIntegerOverflow=on  InputSameDT=on  OutDataTypeStr=Inherit: Same as first input
  Product1 : Product  Orientation=left  OutDataType=sfix(16)  OutScaling=2^0  SaturateOnIntegerOverflow=on  InputSameDT=on  OutDataTypeStr=Inherit: Same as first input
  Sign : Signum  Orientation=left
  Torque radius * # of surfaces : Gain  Orientation=left  Gain=rtq*Nf  ParameterDataType=sfix(16)  ParameterScaling=2^0  OutDataType=sfix(16)  OutScaling=2^0  SaturateOnIntegerOverflow=on  OutDataTypeStr=Inherit: Same as input  ParamDataTypeStr=Inherit: Same as input
  mu : Lookup  Orientation=left  InputValues=mutable(:,1)  Table=mutable(:,2)  OutDataType=sfix(16)  OutScaling=2^0  SaturateOnIntegerOverflow=on
  Clutch : PMIOPort  Orientation=down  Port=1  Side=Right
  tag scope: Slip24=global, Torque24=global
  wires:
  Force/1 -> Torque radius * # of surfaces/1
  mu/1 -> Product/1
  Product1/1 -> Joint Stiction Actuator/2
  Constant/1 -> Joint Stiction Actuator/1
  Product/1 -> Gain/1, Joint Stiction Actuator/5  "Capacity"
  Torque radius * # of surfaces/1 -> Product/2
  Sign/1 -> Product1/1
  Gain/1 -> Joint Stiction Actuator/3, Product1/2
  Joint Sensor/1 -> Abs/1, Sign/1, [Slip24]  "Slip"
  Abs/1 -> mu/1
  Joint Sensor/2 -> Joint Stiction Actuator/4, [Torque24]  "Computed torque"
  connections:
  Ground/RConn1 -- Clutch 24/LConn1
  Clutch/RConn1 -- Clutch 24/RConn1
  Clutch 24/RConn2 -- Joint Sensor/LConn1
  Joint Stiction Actuator/RConn1 -- Clutch 24/LConn2

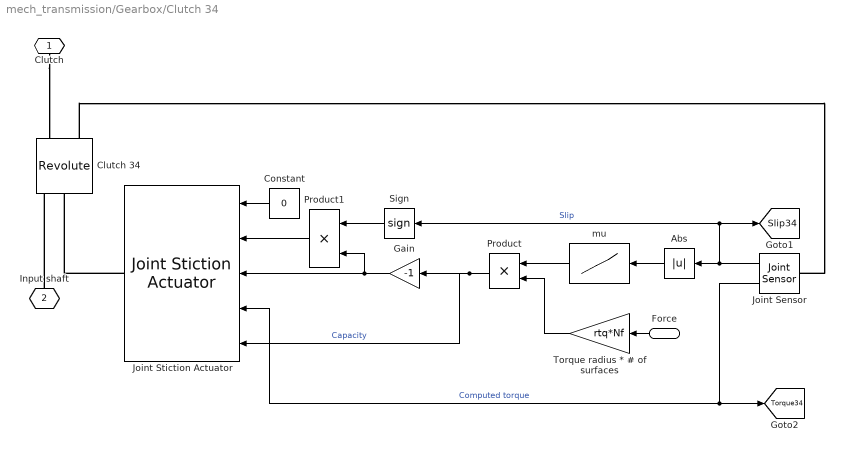
== system mech_transmission/Gearbox/Clutch 34 ==
  Force : Inport  Orientation=left  OutDataType=sfix(16)  OutScaling=2^0
  Abs : Abs  Orientation=left  ZeroCross=off  SaturateOnIntegerOverflow=on
  Clutch 34 : mblibv1/Joints/Revolute  Tag=Factory generic  Description=Mechanical Blockset  Orientation=up  DialogController=MECH.DynMechDlgSource  PhysicalDomain=mechanical  SubClassName=Unknown  LeftPortType=blob  RightPortType=blob  LConnTagsString=__newl0|SA1|SA2  RConnTagsString=__newr0|SA1  NumSAPorts=3  CutJoint=on  MarkAsCut=off  Primitives=revolute  PrimitiveProps=R1$WORLD$[0 0 1]$revolute  DialogClass=JointBlock  R1Axis=[0 0 1]
  Constant : Constant  Orientation=left  Value=0  OutDataType=sfix(16)  OutScaling=2^0
  Gain : Gain  Orientation=left  Gain=-1  ParameterDataType=sfix(16)  ParameterScaling=2^0  OutDataType=sfix(16)  OutScaling=2^0  SaturateOnIntegerOverflow=on  OutDataTypeStr=Inherit: Same as input  ParamDataTypeStr=Inherit: Same as input
  Joint Sensor : mblibv1/Sensors &  Actuators/Joint Sensor  Description=Mechanical Blockset  Orientation=left  DialogController=MECH.DynMechDlgSource  SystemSampleTime=-1  PhysicalDomain=Mechanical  PortType=blob  Muxed=off  Pose=off  Angle=off  AngleUnits=deg  ArcVelocity=on  ArcVelocityUnits=rad/s  ArcAcceleration=off  ArcAccelerationUnits=deg/s^2  CoordPosition=on  CoordPositionUnits=m  Velocity=off  VelocityUnits=m/s  Acceleration=off  AccelerationUnits=m/s^2  Quaternion=on  QuaternionDT=off  QuaternionDDT=off  QuaternionUnits=off  OutputVector=[ 1 1 ]  ActiveIO=on  Width=2  DialogClass=MechanicalSensorBlock  Primitive=R1  Force=off  ForceUnits=N  Torque=on  TorqueUnits=N-m  ReferenceFrame=Absolute (INERTIAL)  ReactionSensedSide=Base  ReactionReferenceFrame=Absolute (World)  ReactionForce=off  ReactionForceUnits=N  ReactionMoment=off  ReactionMomentUnits=N-m
  Joint Stiction Actuator : mblibv1/Sensors &  Actuators/Joint Stiction Actuator  Description=Mechanical Blockset  Orientation=left  DialogController=MECH.DynMechDlgSource  SystemSampleTime=-1  PhysicalDomain=Mechanical  PortType=blob  ActuationStyle=Force  AngleUnits=deg  ArcVelocityUnits=deg/s  ArcAccelerationUnits=deg/s^2  CoordPositionUnits=m  VelocityUnits=m/s  AccelerationUnits=m/s^2  ForceUnits=N  TorqueUnits=N-m  ActiveIO=on  Width=5  DialogClass=EventActuatorBlock  Primitive=R1  FrictionalForceUnits=N-m  ExternalForceUnits=N-m  FrictionalTorqueUnits=N-m  ExternalTorqueUnits=N-m  LockingTolerance=1e-3
  Product : Product  Orientation=left  OutDataType=sfix(16)  OutScaling=2^0  SaturateOnIntegerOverflow=on  InputSameDT=on  OutDataTypeStr=Inherit: Same as first input
  Product1 : Product  Orientation=left  OutDataType=sfix(16)  OutScaling=2^0  SaturateOnIntegerOverflow=on  InputSameDT=on  OutDataTypeStr=Inherit: Same as first input
  Sign : Signum  Orientation=left
  Torque radius * # of surfaces : Gain  Orientation=left  Gain=rtq*Nf  ParameterDataType=sfix(16)  ParameterScaling=2^0  OutDataType=sfix(16)  OutScaling=2^0  SaturateOnIntegerOverflow=on  OutDataTypeStr=Inherit: Same as input  ParamDataTypeStr=Inherit: Same as input
  mu : Lookup  Orientation=left  InputValues=mutable(:,1)  Table=mutable(:,2)  OutDataType=sfix(16)  OutScaling=2^0  SaturateOnIntegerOverflow=on
  Clutch : PMIOPort  Orientation=down  Port=1  Side=Right
  Input shaft : PMIOPort  Orientation=up  Port=2  Side=Left
  tag scope: Slip34=global, Torque34=global
  wires:
  Joint Sensor/2 -> Joint Stiction Actuator/4, [Torque34]  "Computed torque"
  Abs/1 -> mu/1
  Joint Sensor/1 -> Abs/1, [Slip34], Sign/1  "Slip"
  Gain/1 -> Product1/2, Joint Stiction Actuator/3
  Sign/1 -> Product1/1
  Torque radius * # of surfaces/1 -> Product/2
  Product/1 -> Gain/1, Joint Stiction Actuator/5  "Capacity"
  Constant/1 -> Joint Stiction Actuator/1
  Product1/1 -> Joint Stiction Actuator/2
  mu/1 -> Product/1
  Force/1 -> Torque radius * # of surfaces/1
  connections:
  Clutch 34/RConn2 -- Joint Sensor/LConn1
  Joint Stiction Actuator/RConn1 -- Clutch 34/LConn2
  Clutch/RConn1 -- Clutch 34/RConn1
  Input shaft/RConn1 -- Clutch 34/LConn1

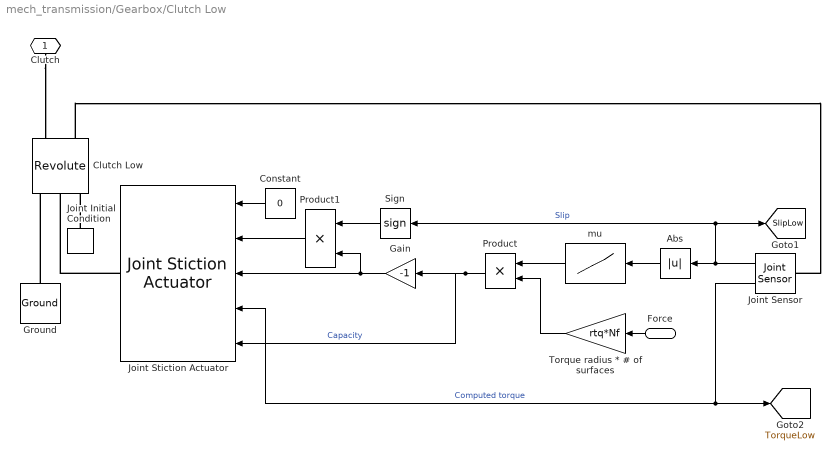
== system mech_transmission/Gearbox/Clutch Low ==
  Force : Inport  Orientation=left  OutDataType=sfix(16)  OutScaling=2^0
  Abs : Abs  Orientation=left  ZeroCross=off  SaturateOnIntegerOverflow=on
  Clutch Low : mblibv1/Joints/Revolute  Tag=Factory generic  Description=Mechanical Blockset  Orientation=up  DialogController=MECH.DynMechDlgSource  PhysicalDomain=mechanical  SubClassName=Unknown  LeftPortType=blob  RightPortType=blob  LConnTagsString=__newl0|SA1|SA2  RConnTagsString=__newr0|SA1  NumSAPorts=3  CutJoint=on  MarkAsCut=off  Primitives=revolute  PrimitiveProps=R1$WORLD$[0 0 1]$revolute  DialogClass=JointBlock  R1Axis=[0 0 1]
  Constant : Constant  Orientation=left  Value=0  OutDataType=sfix(16)  OutScaling=2^0
  Gain : Gain  Orientation=left  Gain=-1  ParameterDataType=sfix(16)  ParameterScaling=2^0  OutDataType=sfix(16)  OutScaling=2^0  SaturateOnIntegerOverflow=on  OutDataTypeStr=Inherit: Same as input  ParamDataTypeStr=Inherit: Same as input
  Ground : mblibv1/Bodies/Ground  Orientation=up  DialogController=MECH.DynMechDlgSource  SystemSampleTime=-1  LeftPortType=env  RightPortType=workingframe  PhysicalDomain=Mechanical  DialogClass=GroundBlock  CoordPosition=[0 0 0]  CoordPositionUnits=m  StateVectorMgrId=-1  MachineId=[0 0]  ShowEnvPort=off
  Joint Initial Condition : mblibv1/Sensors &  Actuators/Joint Initial Condition  Description=Mechanical Blockset  Orientation=up  DialogController=MECH.DynMechDlgSource  SystemSampleTime=-1  PhysicalDomain=Mechanical  DialogClass=InitialConditionBlock  Primitive=R1  CoordPosition=0.0  Velocity=0.0  AngleUnits=rad  ArcVelocityUnits=rad/s  CoordPositionUnits=m  VelocityUnits=m/s  InitialConditions=P1$false$0$m$rad$0$m/s$rad/s#P2$false$0$m$rad$0$m/s$rad/s#P3$false$0$m$rad$0$m/s$rad/s#R1$true$0.0$m$rad$0.0$m/s$rad/s#R2$false$0$m$rad$0$m/s$rad/s#R3$false$0$m$rad$0$m/s$rad/s#S$false$0$m$rad$0$m/s$rad/s  P1PIC=0  P1VIC=0  P2PIC=0  P2VIC=0  P3PIC=0  P3VIC=0  R1PIC=0.0  R1VIC=0.0  R2PIC=0  R2VIC=0  R3PIC=0  R3VIC=0  SPIC=0  SVIC=0
  Joint Sensor : mblibv1/Sensors &  Actuators/Joint Sensor  Description=Mechanical Blockset  Orientation=left  DialogController=MECH.DynMechDlgSource  SystemSampleTime=-1  PhysicalDomain=Mechanical  PortType=blob  Muxed=off  Pose=off  Angle=off  AngleUnits=deg  ArcVelocity=on  ArcVelocityUnits=rad/s  ArcAcceleration=off  ArcAccelerationUnits=deg/s^2  CoordPosition=on  CoordPositionUnits=m  Velocity=off  VelocityUnits=m/s  Acceleration=off  AccelerationUnits=m/s^2  Quaternion=on  QuaternionDT=off  QuaternionDDT=off  QuaternionUnits=off  OutputVector=[ 1 1 ]  ActiveIO=on  Width=2  DialogClass=MechanicalSensorBlock  Primitive=R1  Force=off  ForceUnits=N  Torque=on  TorqueUnits=N-m  ReferenceFrame=Absolute (INERTIAL)  ReactionSensedSide=Base  ReactionReferenceFrame=Absolute (World)  ReactionForce=off  ReactionForceUnits=N  ReactionMoment=off  ReactionMomentUnits=N-m
  Joint Stiction Actuator : mblibv1/Sensors &  Actuators/Joint Stiction Actuator  Description=Mechanical Blockset  Orientation=left  DialogController=MECH.DynMechDlgSource  SystemSampleTime=-1  PhysicalDomain=Mechanical  PortType=blob  ActuationStyle=Force  AngleUnits=deg  ArcVelocityUnits=deg/s  ArcAccelerationUnits=deg/s^2  CoordPositionUnits=m  VelocityUnits=m/s  AccelerationUnits=m/s^2  ForceUnits=N  TorqueUnits=N-m  ActiveIO=on  Width=5  DialogClass=EventActuatorBlock  Primitive=R1  FrictionalForceUnits=N-m  ExternalForceUnits=N-m  FrictionalTorqueUnits=N-m  ExternalTorqueUnits=N-m  LockingTolerance=1e-3
  Product : Product  Orientation=left  OutDataType=sfix(16)  OutScaling=2^0  SaturateOnIntegerOverflow=on  InputSameDT=on  OutDataTypeStr=Inherit: Same as first input
  Product1 : Product  Orientation=left  OutDataType=sfix(16)  OutScaling=2^0  SaturateOnIntegerOverflow=on  InputSameDT=on  OutDataTypeStr=Inherit: Same as first input
  Sign : Signum  Orientation=left
  Torque radius * # of surfaces : Gain  Orientation=left  Gain=rtq*Nf  ParameterDataType=sfix(16)  ParameterScaling=2^0  OutDataType=sfix(16)  OutScaling=2^0  SaturateOnIntegerOverflow=on  OutDataTypeStr=Inherit: Same as input  ParamDataTypeStr=Inherit: Same as input
  mu : Lookup  Orientation=left  InputValues=mutable(:,1)  Table=mutable(:,2)  OutDataType=sfix(16)  OutScaling=2^0  SaturateOnIntegerOverflow=on
  Clutch : PMIOPort  Orientation=down  Port=1  Side=Right
  tag scope: SlipLow=global, TorqueLow=global
  wires:
  Joint Sensor/2 -> [TorqueLow], Joint Stiction Actuator/4  "Computed torque"
  Abs/1 -> mu/1
  Joint Sensor/1 -> Abs/1, [SlipLow], Sign/1  "Slip"
  Gain/1 -> Product1/2, Joint Stiction Actuator/3
  Sign/1 -> Product1/1
  Torque radius * # of surfaces/1 -> Product/2
  Product/1 -> Gain/1, Joint Stiction Actuator/5  "Capacity"
  Constant/1 -> Joint Stiction Actuator/1
  Product1/1 -> Joint Stiction Actuator/2
  mu/1 -> Product/1
  Force/1 -> Torque radius * # of surfaces/1
  connections:
  Clutch Low/RConn2 -- Joint Sensor/LConn1
  Joint Stiction Actuator/RConn1 -- Clutch Low/LConn2
  Clutch/RConn1 -- Clutch Low/RConn1
  Ground/RConn1 -- Clutch Low/LConn1
  Joint Initial Condition/RConn1 -- Clutch Low/LConn3
